simulink model "SkywalkerX8_TrimAndLinearize"  (R2018a)
settings: Solver=FixedStepAuto  StartTime=0.0  StopTime=0.789  FixedStep=0.001  RelTol=1e-3
libraries: aerolibatmos2 x1
settings Model: Creator=David  LastModifiedBy=David

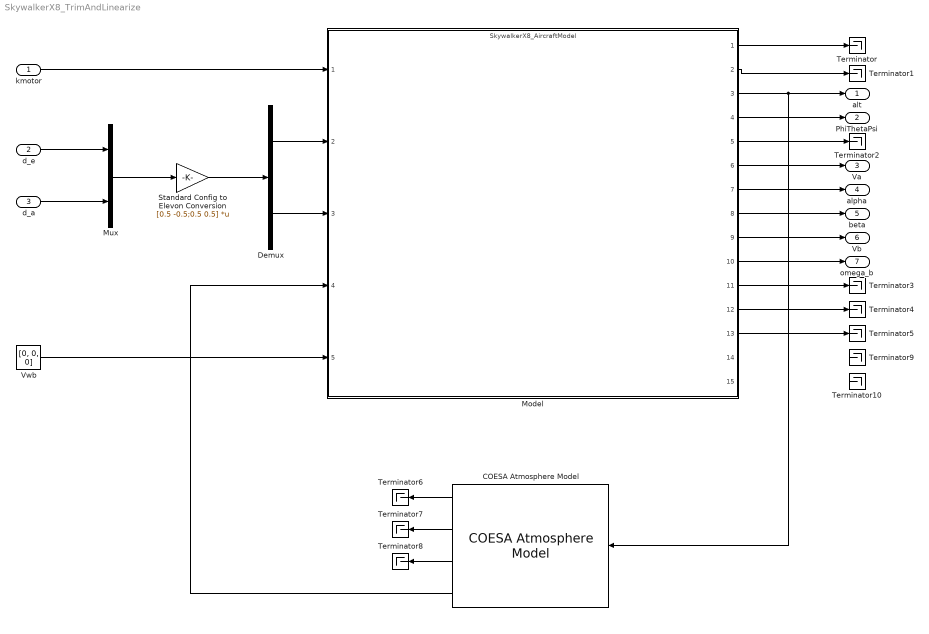
== system SkywalkerX8_TrimAndLinearize ==
  kmotor : Inport
  d_e : Inport  Port=2
  d_a : Inport  Port=3
  COESA Atmosphere Model : aerolibatmos2/COESA Atmosphere Model  units=Metric (MKS)  spec=1976 COESA-extended U.S. Standard Atmosphere  model=Profile  profile_var=High temperature  profile_percent=1%  profile_alt=5 km (16404 ft)  envelope_var=High temperature  envelope_percent=1%  action=None
  Demux : Demux  Outputs=2
  Model : ModelReference  ModelNameDialog=SkywalkerX8_AircraftModel  ModelReferenceVersion=1.171
      mask Display:
      | image('C:\MATLAB\masters\icons\Skywalker Main Block Icon.png', 'center')
      | 
      | color('cyan')
      | 
      | port_label('input', 1, 'k_{motor} (Unitless)', 'texmode', 'on')
      | port_label('input', 2, '\delta_{er} (rad)', 'texmode', 'on')
      | port_label('input', 3, '\delta_{el} (rad)', 'texmode', 'on')
      | port_label('input', 4, '\rho (kg/m^3)', 'texmode', 'on')
      | port_label('input', 5, '{\bf V_w^b} (m/s)', 'texmode', 'on')
      | 
      | port_label('output', 1, '{\bf V_e} (m/s)', 'texmode', 'on')
      | port_label('output', 2, '{\bf X_e} (m)', 'texmode', 'on')
      | port_label('output', 3, 'Altitude (m)', 'texmode', 'on')
      | port_label('output', 4, '\phi \theta \psi (rad)', 'texmode', 'on')
      | port_label('output', 5, 'R_{inertial}^{body}', 'texmode', 'on')
      | port_label('output', 6, 'V_a (m/s)', 'texmode', 'on')
      | port_label('output', 7, 'alpha (rad)', 'texmode', 'on')
      | port_label('output', 8, 'beta (rad)', 'texmode', 'on')
      | port_label('output', 9, '{\bf V_b} (m/s)', 'texmode', 'on')
      | port_label('output', 10, '{\bf \omega_b} (rad/s)', 'texmode', 'on')
      | port_label('output', 11, '{\bf \delta\omega_b/\deltat} (rad/s^2)', 'texmode', 'on')
      | port_label('output', 12, '{\bf a_{body}} (m/s^2)', 'texmode', 'on')
      | port_label('output', 13, '{\bf a_{inertial}} (m/s^2)', 'texmode', 'on')
      | port_label('output', 14, '\chi (rad)', 'texmode', 'on')
      | port_label('output', 15, '\chi_c (rad)', 'texmode', 'on')
  Mux : Mux  Inputs=2
  Standard Config to Elevon Conversion : Gain  Gain=[0.5 -0.5;0.5 0.5]  Multiplication=Matrix(K*u)
  Terminator{,1..10} (11 alike) : Terminator
  Vwb : Constant  Value=[0, 0, 0]
  alt : Outport
  PhiThetaPsi : Outport  Port=2
  Va : Outport  Port=3
  alpha : Outport  Port=4
  beta : Outport  Port=5
  Vb : Outport  Port=6
  omega_b : Outport  Port=7
  wires:
  Vwb/1 -> Model/5
  COESA Atmosphere Model/4 -> Model/4
  Demux/2 -> Model/3
  kmotor/1 -> Model/1
  Demux/1 -> Model/2
  Model/1 -> Terminator/1
  Model/2 -> Terminator1/1
  Model/4 -> PhiThetaPsi/1
  Model/5 -> Terminator2/1
  Model/6 -> Va/1
  Model/9 -> Vb/1
  Model/10 -> omega_b/1
  Model/11 -> Terminator3/1
  Model/12 -> Terminator4/1
  Model/13 -> Terminator5/1
  Model/7 -> alpha/1
  Model/8 -> beta/1
  d_e/1 -> Mux/1
  Standard Config to Elevon Conversion/1 -> Demux/1
  d_a/1 -> Mux/2
  Mux/1 -> Standard Config to Elevon Conversion/1
  COESA Atmosphere Model/1 -> Terminator6/1
  COESA Atmosphere Model/2 -> Terminator7/1
  COESA Atmosphere Model/3 -> Terminator8/1
  Model/3 -> COESA Atmosphere Model/1, alt/1
